simulink model "BJStateflow"  (R2012b)
settings: Solver=ode45  StartTime=0.0  StopTime=240  MaxStep=0.1  RelTol=1e-3
settings Model: Creator=fofo  LastModifiedBy=fofo
settings SolverCC: ZeroCrossControl=EnableAll  SolverResetMethod=Robust

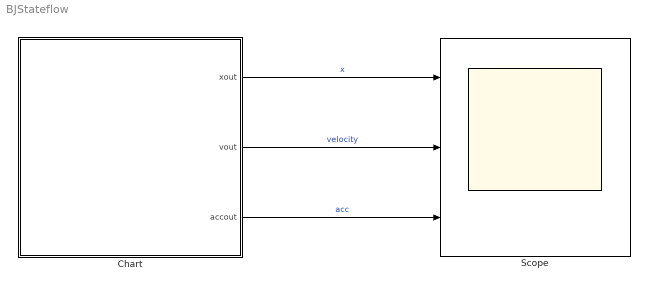
== system BJStateflow ==
  Chart : Stateflow chart  TreatAsAtomicUnit=on
  Scope : Scope  NumInputPorts=3
      settings: ShowLegends=on  TimeRange=240  YMin=-75~-45~-5  YMax=125~40~5
  wires:
  Chart/1(xout) -> Scope/1  "x"
  Chart/2(vout) -> Scope/2  "velocity"
  Chart/3(accout) -> Scope/3  "acc"

== stateflow chart BJStateflow/Chart ==
  settings: updateMethod=CONTINUOUS
  state above0
    en:xout=x;
    du:
    x_dot=v;
    v_dot=g+(-0.05*fabs(v)*v-0.2*v)/m;
    xout=x;
    vout=v;
    accout=g+(-0.05*fabs(v)*v-0.2*v)/m;
  state below0
    en:xout=x;
    du:
    x_dot=v;
    v_dot=g+(-k*x*g-0.05*fabs(v)*v-0.2*v)/m;
    xout=x;
    vout=v;
    accout=g+(-k*x*g-0.05*fabs(v)*v-0.2*v)/m;
  (default) -> above0 : {x=-160;v=0;k=4;g=32;m=160;xout=x;}
  above0 -> below0 : [x>0]
  below0 -> above0 : [x<=0]
  data: value function_input double; absvalue function_output double; xout output double; x local double; v local double; g local double; k local double; m local double; vout output double; accout output double
  data x settings: updateMethod=SF_CONTINUOUS_TIME_DATA
  data v settings: updateMethod=SF_CONTINUOUS_TIME_DATA
  function absvalue=fabs(value):
    | function absvalue=fabs(value)
    | absvalue=abs(value);
    | return;
